simulink subsystem "ReactionWheels_SS"  (R2023a)
settings: Solver=VariableStepAuto  StartTime=0.0  StopTime=10.0  RelTol=1e-3
values from neighbouring files (symbols this model uses):
  Is_matrix = [Iws 0 0; 0 Iws 0; 0 0 Iws]    [WheelSizing_Script.m]
libraries: matrix_library x1
settings Model: Creator=jself  LastModifiedBy=shaniyasingh

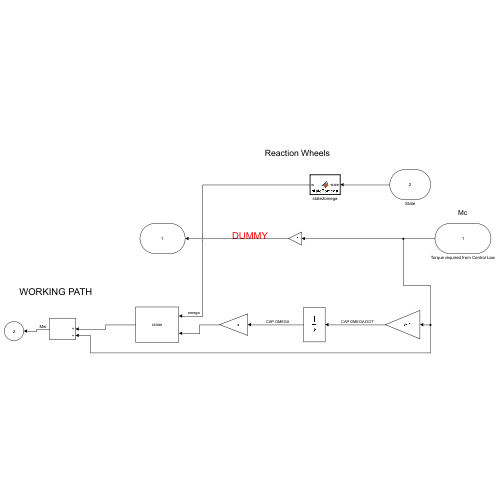
[thumbnail: Simulink's stored preview of the top-level diagram]
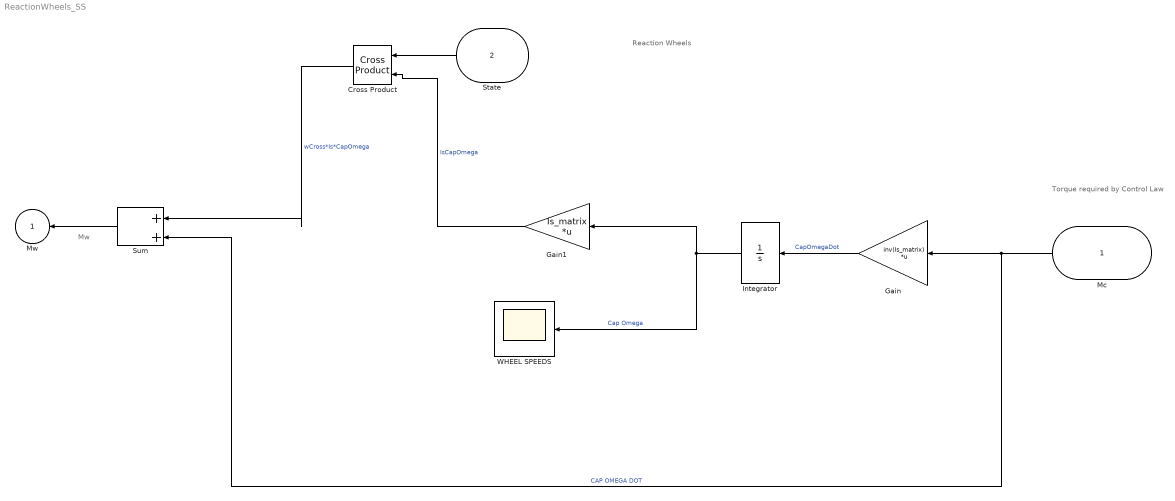
== system ReactionWheels_SS ==
  note: Mw
  note: Torque required by
      | Control Law
  note: Reaction Wheels
  Mc : Inport
  State : Inport  Port=2
  Cross Product : matrix_library/Cross Product
  Gain : Gain  Gain=inv(Is_matrix)  Multiplication=Matrix(K*u)
  Gain1 : Gain  Gain=Is_matrix  Multiplication=Matrix(K*u)
  Integrator : Integrator
  Sum : Sum  Inputs=|++
  WHEEL SPEEDS : Scope
  Mw : Outport
  wires:
  Mc/1 -> Gain/1, Sum/2  "CAP OMEGA DOT"
  Integrator/1 -> WHEEL SPEEDS/1, Gain1/1  "Cap Omega"
  Cross Product/1 -> Sum/1  "wCross*Is*CapOmega"
  Sum/1 -> Mw/1
  Gain/1 -> Integrator/1  "CapOmegaDot"
  Gain1/1 -> Cross Product/2  "IsCapOmega"
  State/1 -> Cross Product/1
